simulink model "linear_dob"  (R2023b)
settings: Solver=ode4  StartTime=0.0  StopTime=10.0  RelTol=1e-3
settings Model: Creator=rodel  LastModifiedBy=rodel
settings DebuggingCC: AlgebraicLoopMsg=none

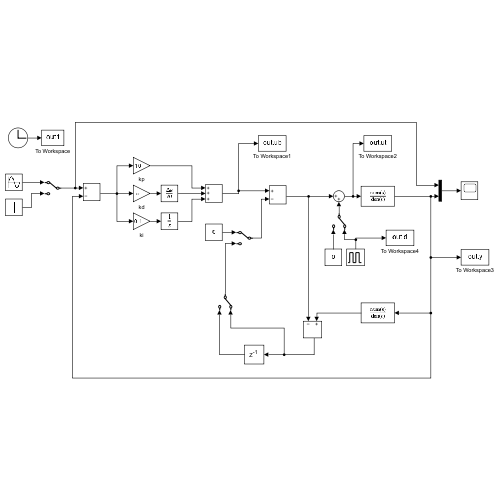
[thumbnail: Simulink's stored preview of the top-level diagram]
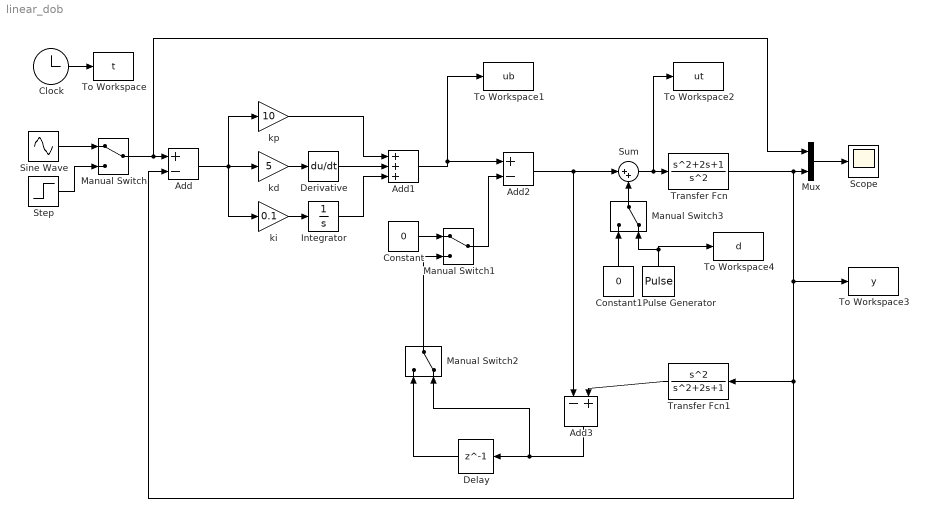
== system linear_dob ==
  Add : Sum  Inputs=+-
  Add1 : Sum  Inputs=+++
  Add2 : Sum  Inputs=+-
  Add3 : Sum  Inputs=-+
  Clock : Clock
  Constant : Constant  Value=0
  Constant1 : Constant  Value=0
  Delay : Delay  DelayLength=1  InitialCondition=0
  Derivative : Derivative
  Integrator : Integrator
  Manual Switch : ManualSwitch
  Manual Switch1 : ManualSwitch
  Manual Switch2 : ManualSwitch  CurrentSetting=0
  Manual Switch3 : ManualSwitch  CurrentSetting=0
  Mux : Mux  Inputs=2
  Pulse Generator : DiscretePulseGenerator  PulseType=Time based  Amplitude=3  Period=1  PulseWidth=20  PhaseDelay=1
  Scope : Scope
  Sine Wave : Sin  SampleTime=0
  Step : Step  Time=0  SampleTime=0  VectorParams1D=off  ZeroCross=off
  Sum : Sum  Inputs=|++
  To Workspace : ToWorkspace  VariableName=t  SampleTime=-1
      settings: Save2DSignal=2-D array (concatenate along first dimension)
  To Workspace1 : ToWorkspace  VariableName=ub  SampleTime=-1
      settings: Save2DSignal=2-D array (concatenate along first dimension)
  To Workspace2 : ToWorkspace  VariableName=ut  SampleTime=-1
      settings: Save2DSignal=2-D array (concatenate along first dimension)
  To Workspace3 : ToWorkspace  VariableName=y  SampleTime=-1
      settings: Save2DSignal=2-D array (concatenate along first dimension)
  To Workspace4 : ToWorkspace  VariableName=d  SampleTime=-1
      settings: Save2DSignal=2-D array (concatenate along first dimension)
  Transfer Fcn : TransferFcn  Numerator=[1 2 1]  Denominator=[1 0 0]
  Transfer Fcn1 : TransferFcn  Numerator=[1 0 0]
  kd : Gain  Gain=5
  ki : Gain  Gain=0.1
  kp : Gain  Gain=10
  wires:
  Clock/1 -> To Workspace/1
  Sine Wave/1 -> Manual Switch/1
  Step/1 -> Manual Switch/2
  Manual Switch/1 -> Add/1, Mux/1
  kd/1 -> Derivative/1
  ki/1 -> Integrator/1
  Derivative/1 -> Add1/2
  kp/1 -> Add1/1
  Integrator/1 -> Add1/3
  Add/1 -> ki/1, kd/1, kp/1
  Add1/1 -> Add2/1, To Workspace1/1
  Constant/1 -> Manual Switch1/1
  Manual Switch1/1 -> Add2/2
  Delay/1 -> Manual Switch2/1
  Add2/1 -> Add3/1, Sum/1
  Add3/1 -> Delay/1, Manual Switch2/2
  Manual Switch2/1 -> Manual Switch1/2
  Manual Switch3/1 -> Sum/2
  Sum/1 -> Transfer Fcn/1, To Workspace2/1
  Mux/1 -> Scope/1
  Transfer Fcn/1 -> Transfer Fcn1/1, Add/2, To Workspace3/1, Mux/2
  Transfer Fcn1/1 -> Add3/2
  Constant1/1 -> Manual Switch3/1
  Pulse Generator/1 -> To Workspace4/1, Manual Switch3/2
